simulink model "vehicle_model_999"  (R2025b)
settings: Solver=ode23tb  StartTime=0.0  StopTime=50  MaxStep=0.001  RelTol=1e-3
values from neighbouring files (symbols this model uses):
  aero_par = struct()    [Load_aero_parameters.m]
  init_r = 0    [Run_this_first.m]
  init_vx = 0    [Run_this_first.m]
  init_vy = 0    [Run_this_first.m]
  m = Par.m    [LapSim_Endurance_final_ts_v2.m]    (also in Lap_Sim_Final_inverse.m = Par.Mass; Lapsim_Endurance_final_ts.m; New_LapSim_final_ts_v1.m = Par.Mass; Torque_vectoring_lookup_table_v3.m = 270)
  Par = struct()    [Load_vehicle_parameters.m]
  sus_par = struct()    [Load_sus_parameters.m]
  TireData = []    [Lapsim_final_for_app.m]
  V_ref = 45    [Run_this_first.m]
undefined symbols (not defined in the file or in its folder): Battery, Brake_Val, HP, Ki_data, Kp_data, Motor, steer_input, Steer_Val, TC_target_slip, Throttle_Val, vx_breakpoints
libraries: simulink x7, autolibshared x2, BatteryEstimators x1
(part 1 of 3)
settings Model: Creator=vishal bhujbal  LastModifiedBy=vishal bhujbal
settings SolverCC: ZeroCrossAlgorithm=Adaptive
settings DebuggingCC: IgnoredZcDiagnostic=none

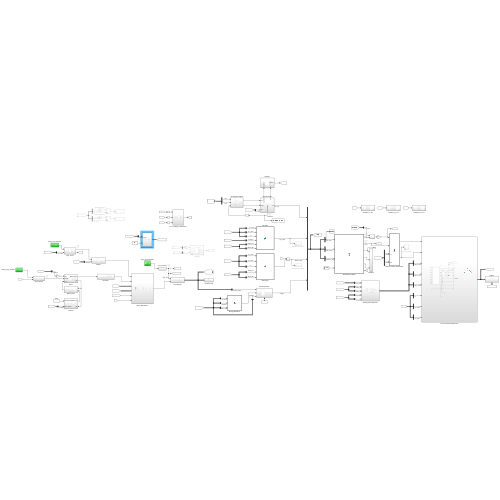
[thumbnail: Simulink's stored preview of the top-level diagram]
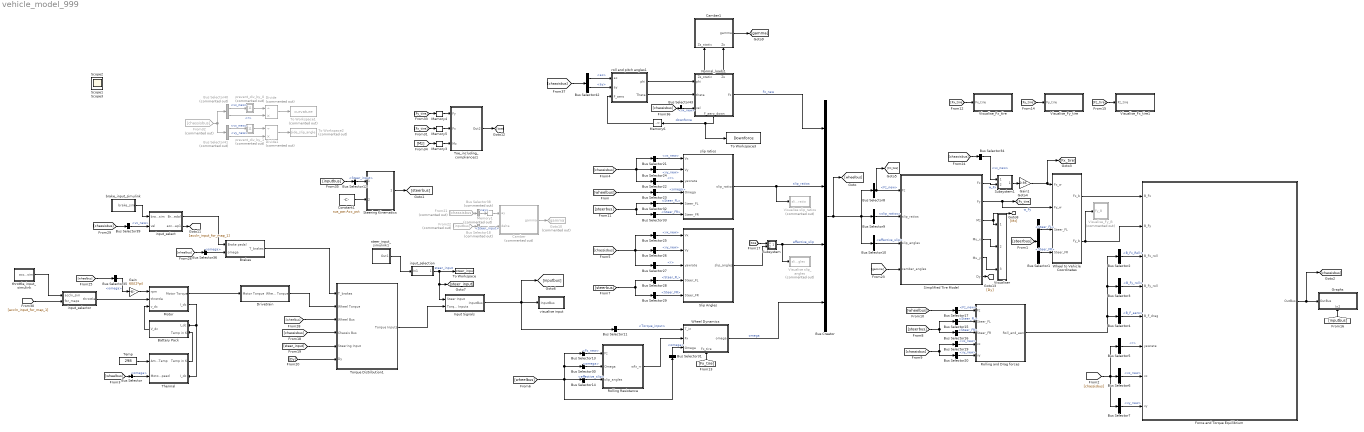
== system vehicle_model_999 ==
  Battery Pack : Subsystem
  Brakes : Subsystem
  Bus Creator : BusCreator  Inputs=4
  Bus Selector{,23,30..31,35..36} (6 alike) : BusSelector  OutputSignals=omega
  Bus Selector1 : BusSelector  OutputSignals=Steer_FL,Steer_FR
  Bus Selector10 : BusSelector  OutputSignals=effective_slip
  Bus Selector11 : BusSelector  OutputSignals=Torque_input
  Bus Selector12 : BusSelector  OutputSignals=Steer_input
  Bus Selector13 : BusSelector  OutputSignals=Fz_new
  Bus Selector14 : BusSelector  OutputSignals=effective_slip
  Bus Selector15 : BusSelector  OutputSignals=Steer_FL
  Bus Selector16 : BusSelector  OutputSignals=Steer_FR
  Bus Selector17 : BusSelector  OutputSignals=Fz_new
  Bus Selector18 : BusSelector  Commented=on  OutputSignals=Steer_input
  Bus Selector{6,19,21,25,34,39,43} (7 alike) : BusSelector  OutputSignals=vx_new
  Bus Selector2 : BusSelector  OutputSignals=B_Fx_Roll
  Bus Selector{7,20,24,26} (4 alike) : BusSelector  OutputSignals=vy_new
  Bus Selector22 : BusSelector  OutputSignals=r
  Bus Selector27 : BusSelector  OutputSignals=r
  Bus Selector28 : BusSelector  OutputSignals=Steer_FL
  Bus Selector29 : BusSelector  OutputSignals=Steer_FR
  Bus Selector3 : BusSelector  OutputSignals=B_Fy_roll
  Bus Selector32 : BusSelector  OutputSignals=Steer_FL
  Bus Selector33 : BusSelector  OutputSignals=Steer_FR
  Bus Selector38 : BusSelector  Commented=on  OutputSignals=ay
  Bus Selector4 : BusSelector  OutputSignals=B_F_aero
  Bus Selector40 : BusSelector  Commented=on  OutputSignals=vx_new,r
  Bus Selector41 : BusSelector  Commented=on  OutputSignals=vx_new,vy_new
  Bus Selector42 : BusSelector  OutputSignals=ax,ay
  Bus Selector5 : BusSelector  OutputSignals=r
  Bus Selector8 : BusSelector  OutputSignals=Fz_new
  Bus Selector9 : BusSelector  OutputSignals=slip_ratios
  Camber : Subsystem  Commented=on
  Camber1 : Subsystem
      settings: PortSchema="{\"entries\":[{\"content\":{\"sides\":[{\"content\":{},\"type\":\"ConnectorPlacement.EquallySpacedRectSide\",\"uuid\":\"3195d381-be28-49da-8fb0-abb81acde47d\"},{\"content\":{\"connectorIds\":[\"Out1\"],\"side\":\"RIGHT\"},\"type\":\"ConnectorPlacement.EquallySpacedRectSide\",\"uuid\":\"ee555968-c3bd-4b66-9d31-d91577019264\"},{\"content\":{\"side\":\"TOP\"},\"type\":\"ConnectorPlacement.EquallySpacedRectSide\",\"uuid\":\"4eacfe39-9434-48f3-a8a4-10327827cbf3\"},{\"content\":{\"connectorIds\":[\"In1\",\"In2\"],\"side\":\"BOTTOM\"},\"type\":\"ConnectorPlacement.EquallySpacedRectSide\",\"uuid\":\"1ccd728a-99da-4160-890d-6a6cfd29e494\"}]},\"type\":\"ConnectorPlacement.EquallySpacedConnector\",\"uuid\":\"ab2607e9-2e18-4a39-9990-bbd46a8a23e6\"}],\"packageUris\":[\"http://schema.mathworks.com/mf0/Connector/R2020b\"],\"version\":\"1.0\"}"
  Constant1 : Constant  Value=sus_par.Acc_pct
  Divide : Product  Commented=on  Inputs=/*
  Divide1 : Product  Commented=on  Inputs=/*
  Drivetrain : Subsystem
  Force and Torque Equilibrium : Subsystem
  From21 : From  Commented=on  GotoTag=chassisbus
  From22 : From  Commented=on  GotoTag=inputbus
  From32 : From  Commented=on  GotoTag=chassisbus
  Gain : Gain  Gain=60/(2*pi)
  Gain1 : Gain  Gain=0.95
  Goto10 : Goto  Commented=on  GotoTag=gamma
  Graphs : Subsystem
      settings: PortSchema="{\"entries\":[{\"content\":{\"sides\":[{\"content\":{\"connectorIds\":[\"In1\"]},\"type\":\"ConnectorPlacement.EquallySpacedRectSide\",\"uuid\":\"0d7f1a6c-503e-4c9f-90e9-70f717dd7dfc\"},{\"content\":{\"side\":\"RIGHT\"},\"type\":\"ConnectorPlacement.EquallySpacedRectSide\",\"uuid\":\"62097468-b066-4e29-8f99-7427d14bee77\"},{\"content\":{\"side\":\"TOP\"},\"type\":\"ConnectorPlacement.EquallySpacedRectSide\",\"uuid\":\"2a3f381e-a201-4804-99b7-77b73504b102\"},{\"content\":{\"connectorIds\":[\"In2\"],\"side\":\"BOTTOM\"},\"type\":\"ConnectorPlacement.EquallySpacedRectSide\",\"uuid\":\"dae5de0a-879c-4844-a347-7056417d054f\"}]},\"type\":\"ConnectorPlacement.EquallySpacedConnector\",\"uuid\":\"aa2835d0-6748-4566-adf9-84e8214dd5a8\"}],\"packageUris\":[\"http://schema.mathworks.com/mf0/Connector/R2020b\"],\"version\":\"1.0\"}"
  Input Signals : Subsystem
  Memory1 : Memory  Commented=on
  Memory3 : Memory
  Memory4 : Memory
  Memory5 : Memory
  Memory6 : Memory  InheritSampleTime=on
  Motor : Subsystem
  Normal_loads1 : Subsystem
      settings: PortSchema="{\"entries\":[{\"content\":{\"sides\":[{\"content\":{\"connectorIds\":[\"In1\",\"In2\",\"In3\"]},\"type\":\"ConnectorPlacement.EquallySpacedRectSide\",\"uuid\":\"5b7db607-33bd-4d54-b958-3aa960e46147\"},{\"content\":{\"connectorIds\":[\"Out1\"],\"side\":\"RIGHT\"},\"type\":\"ConnectorPlacement.EquallySpacedRectSide\",\"uuid\":\"c12df481-c511-4c4c-afb1-8a5812ce44a5\"},{\"content\":{\"connectorIds\":[\"Out3\",\"Out4\"],\"side\":\"TOP\"},\"type\":\"ConnectorPlacement.EquallySpacedRectSide\",\"uuid\":\"2c6024fe-fe45-4ba9-a61f-594b86562523\"},{\"content\":{\"connectorIds\":[\"Out2\"],\"side\":\"BOTTOM\"},\"type\":\"ConnectorPlacement.EquallySpacedRectSide\",\"uuid\":\"099189a9-186d-4ac0-a0af-1ec3a070ea03\"}]},\"type\":\"ConnectorPlacement.EquallySpacedConnector\",\"uuid\":\"81c2e338-68e5-401a-bb4f-0a973fbf41e6\"}],\"packageUris\":[\"http://schema.mathworks.com/mf0/Connector/R2020b\"],\"version\":\"1.0\"}"
  Rolling Resistance : MATLAB Function  TreatAsAtomicUnit=on
  Rolling and Drag forces : Subsystem
  Simplified Tire Model : MATLAB Function  TreatAsAtomicUnit=on
  Slip Angles : MATLAB Function  TreatAsAtomicUnit=on
  Steering Kinematics : Subsystem
  Subsystem : Subsystem
  Subsystem1 : Subsystem
  Temp : Constant  Value=298
  Thermal : Subsystem
      settings: PortSchema="{\"entries\":[{\"content\":{\"sides\":[{\"content\":{\"connectorIds\":[\"In1\",\"In2\"]},\"type\":\"ConnectorPlacement.EquallySpacedRectSide\",\"uuid\":\"a459bc8b-3545-425c-aaae-78f1ff6585f2\"},{\"content\":{\"connectorIds\":[\"Out1\",\"In3\"],\"side\":\"RIGHT\"},\"type\":\"ConnectorPlacement.EquallySpacedRectSide\",\"uuid\":\"31a206fc-68ac-4231-a8cf-74658368026e\"},{\"content\":{\"side\":\"TOP\"},\"type\":\"ConnectorPlacement.EquallySpacedRectSide\",\"uuid\":\"62e9ed2c-7fdb-44da-8c66-64d12a4ececa\"}]},\"type\":\"ConnectorPlacement.EquallySpacedConnector\",\"uuid\":\"e39d97fd-83d5-4a03-8b08-8c3e142a294f\"}],\"packageUris\":[\"http://schema.mathworks.com/mf0/Connector/R2020b\"],\"version\":\"1.0\"}"
  To Workspace : ToWorkspace  VariableName=steer_input  SaveFormat=Timeseries  SampleTime=-1
  To Workspace1 : ToWorkspace  Commented=on  VariableName=curvature  SaveFormat=Timeseries  SampleTime=-1
  To Workspace2 : ToWorkspace  Commented=on  VariableName=side_slip_angle  SaveFormat=Timeseries  SampleTime=-1
  To Workspace3 : ToWorkspace  VariableName=Downforce  SaveFormat=Timeseries  SampleTime=-1
  Toe_including_compliances1 : Subsystem
  Torque Distribution1 : Subsystem
  Visualise slip_angles : Subsystem  Commented=on
  Visualise slip_ratios : Subsystem  Commented=on
  Visualise_Fx_tire : Subsystem
  Visualise_Fx_tire1 : Subsystem
  Visualise_Fy_B : Subsystem  Commented=on
  Visualise_Fy_tire : Subsystem
  Visualiser : Subsystem
  Wheel Dynamics : Subsystem
      settings: PortSchema="{\"entries\":[{\"content\":{\"sides\":[{\"content\":{\"connectorIds\":[\"In1\",\"In2\",\"In3\"]},\"type\":\"ConnectorPlacement.EquallySpacedRectSide\",\"uuid\":\"f2e918e6-c6f6-4ec9-89f3-e2543a6374fd\"},{\"content\":{\"connectorIds\":[\"Out1\"],\"side\":\"RIGHT\"},\"type\":\"ConnectorPlacement.EquallySpacedRectSide\",\"uuid\":\"be700f5f-5cf3-4eec-a6f7-872bb7cd40f6\"},{\"content\":{\"side\":\"TOP\"},\"type\":\"ConnectorPlacement.EquallySpacedRectSide\",\"uuid\":\"c4f49273-9888-4d11-a98e-35dc6f585916\"},{\"content\":{\"connectorIds\":[\"In4\"],\"side\":\"BOTTOM\"},\"type\":\"ConnectorPlacement.EquallySpacedRectSide\",\"uuid\":\"8d2e7982-4362-4abb-b8fe-c155beeed1bc\"}]},\"type\":\"ConnectorPlacement.EquallySpacedConnector\",\"uuid\":\"4d6dafa1-905e-4e38-a48b-73a98e690073\"}],\"packageUris\":[\"http://schema.mathworks.com/mf0/Connector/R2020b\"],\"version\":\"1.0\"}"
  Wheel to Vehicle Coordinates : MATLAB Function  TreatAsAtomicUnit=on
  brake_input_simulink : Subsystem
  input_select : Subsystem
  input_selection : Subsystem
  input_selector : Subsystem
  prevent_div_by_0 : Subsystem  Commented=on
  prevent_div_by_1 : Subsystem  Commented=on
  roll and pitch angles1 : Subsystem
  slip ratios : MATLAB Function  TreatAsAtomicUnit=on
  steer_input_simulink1 : Subsystem
  throttle_input_simulink : Subsystem
  visualise input : Subsystem
  Scope1 : Scope
      settings: ActiveDisplayYMinimum=-36.556875  ActiveDisplayYMaximum=329.01187500000003  DataLoggingVariableName=ScopeData7
  Scope2 : Scope
      settings: ActiveDisplayYMinimum=-33.26675625  ActiveDisplayYMaximum=299.40080625000007  DataLoggingVariableName=ScopeData9
  Scope3 : Scope
      settings: ActiveDisplayYMinimum=-1  ActiveDisplayYMaximum=1  DataLoggingVariableName=ScopeData10
  wires:
  [toe] -> Subsystem/1(toe)
  [Fy_tire] -> Visualise_Fy_tire/1(Fy_tire)
  From22/1 -> Bus Selector18/1
  Bus Selector33/1 -> slip ratios/6(Steer_FR)  "<Steer_FR>"
  Subsystem/1(Out1) -> Bus Creator/3, Visualise slip_angles/1(slip_angles)  "effective_slip"
  Bus Selector41/2 -> Divide1/2  "<vy_new>"
  Bus Selector15/1 -> Rolling and Drag forces/2(Steer_FL)  "<Steer_FL>"
  [wheelbus] -> Bus Selector35/1
  Input Signals/1(InputBus) -> [inputbus], visualise input/1(InputBus), Bus Selector11/1
  [chassisbus] -> Bus Selector27/1, Bus Selector26/1, Bus Selector25/1
  input_select/2(accln_for_map1) -> [accln_input_for_map_1]
  Bus Selector41/1 -> prevent_div_by_1/1(In1)  "<vx_new>"
  Bus Selector1/1 -> Wheel to Vehicle Coordinates/3(Steer_FL)  "<Steer_FL>"
  Motor/1(Motor Torque) -> Drivetrain/1(Motor Torque)
  Bus Selector27/1 -> Slip Angles/3(yawrate)  "<r>"
  [steerbus] -> Bus Selector33/1, Bus Selector32/1
  Simplified Tire Model/2(Fy) -> Wheel to Vehicle Coordinates/2(Fy_w), [Fy_tire]  "w_Fy"
  Bus Selector11/1 -> Wheel Dynamics/1(T_in)  "<Torque_input>"
  prevent_div_by_0/1(Out1) -> Divide/1
  Bus Selector26/1 -> Slip Angles/2(Vy)  "<vy_new>"
  [inputbus] -> Graphs/2(In2)
  Bus Selector14/1 -> Rolling Resistance/3(slip_angles)  "<effective_slip>"
  [chassisbus] -> Bus Selector39/1
  Bus Selector25/1 -> Slip Angles/1(Vx)  "<vx_new>"
  Temp/1 -> Thermal/1(Ambient Temp)
  [accln_input_for_map_1] -> input_selector/2(for_maps)
  Bus Selector30/1 -> Rolling Resistance/2(Omega)  "<omega>"
  Gain/1 -> Motor/1(rpm)
  Divide/1 -> To Workspace1/1
  Rolling and Drag forces/1(Roll_and_aero) -> Bus Selector2/1, Bus Selector3/1, Bus Selector4/1
  Bus Selector20/1 -> Rolling and Drag forces/5(vy)  "<vy_new>"
  input_selection/1(Steer Input) -> Input Signals/1(Steer Input), [steer_input], To Workspace/1  "steer_input"
  [steerbus] -> Bus Selector1/1
  Simplified Tire Model/4(Mu_x) -> Visualiser/2(mu_x)
  Force and Torque Equilibrium/1(OutBus) -> Graphs/1(OutBus), [chassisbus]
  Drivetrain/1(Wheel Torque) -> Torque Distribution1/2(Wheel Torque)
  Bus Selector5/1 -> Force and Torque Equilibrium/6(yawrate)  "<r>"
  Bus Selector35/1 -> Gain/1  "<omega>"
  Rolling Resistance/1(wFx_rr) -> Wheel Dynamics/2(Fx)
  Bus Selector18/1 -> Camber/2(delta)  "<Steer_input>"
  Bus Selector24/1 -> slip ratios/2(Vy)  "<vy_new>"
  Bus Selector9/1 -> Simplified Tire Model/2(slip_ratios)  "<slip_ratios>"
  Bus Creator/1 -> Bus Selector10/1, Bus Selector8/1, Bus Selector9/1, [wheelbus]
  [chassisbus] -> Bus Selector34/1
  Camber/1(gamma) -> Goto10/1
  Battery Pack/1(V_dc) -> Motor/3(v_dc)
  Bus Selector16/1 -> Rolling and Drag forces/3(Steer_FR)  "<Steer_FR>"
  Bus Selector22/1 -> slip ratios/3(yawrate)  "<r>"
  Bus Selector17/1 -> Rolling and Drag forces/1(Fz)  "<Fz_new>"
  [gamma] -> Simplified Tire Model/4(camber_angles)
  [chassisbus] -> Bus Selector22/1, Bus Selector24/1, Bus Selector21/1
  [steerbus] -> Bus Selector29/1, Bus Selector28/1
  Bus Selector10/1 -> Simplified Tire Model/3(slip_angles)  "<effective_slip>"
  input_select/1(Brake pedal) -> Brakes/1(Brake pedal)
  Bus Selector39/1 -> input_select/2(vel)  "<vx_new>"
  Bus Selector19/1 -> Rolling and Drag forces/4(vx)  "<vx_new>"
  [wheelbus] -> Bus Selector13/1, Bus Selector30/1, Bus Selector14/1, Bus Selector31/1
  Bus Selector12/1 -> Steering Kinematics/1(Steer_Input)  "<Steer_input>"
  [wheelbus] -> Bus Selector36/1
  Bus Selector8/1 -> [Fz_tire], Simplified Tire Model/1(Fz)  "<Fz_new>"
  [wheelbus] -> Bus Selector23/1
  [wheelbus] -> Bus Selector17/1
  [Fz_tire] -> Visualise_Fx_tire1/1(Fz_tire)
  Bus Selector40/1 -> prevent_div_by_0/1(In1)  "<vx_new>"
  [Fx_tire] -> Visualise_Fx_tire/1(Fx_tire)
  Bus Selector28/1 -> Slip Angles/4(Steer_FL)  "<Steer_FL>"
  Divide1/1 -> To Workspace2/1
  slip ratios/1(slip_ratios) -> Visualise slip_ratios/1(slip_ratio), Bus Creator/2  "slip_ratios"
  Bus Selector3/1 -> Force and Torque Equilibrium/4(B_Fy_roll)  "<B_Fy_roll>"
  Bus Selector40/2 -> Divide/2  "<r>"
  [inputbus] -> Bus Selector12/1
  Bus Selector21/1 -> slip ratios/1(Vx)  "<vx_new>"
  Brakes/1(T_brakes) -> Torque Distribution1/1(T_brakes)
  Simplified Tire Model/5(Mu_y) -> Visualiser/3(mu_y)
  [chassisbus] -> Bus Selector5/1, Bus Selector6/1, Bus Selector7/1
  Wheel Dynamics/1(omega) -> Bus Creator/4  "omega"
  Slip Angles/1(slip_angles) -> Subsystem/2(slip_angles)
  Bus Selector32/1 -> slip ratios/5(Steer_FL)  "<Steer_FL>"
  Torque Distribution1/1(Torque Inputs) -> Input Signals/2(Torque Inputs)
  Bus Selector34/1 -> Subsystem1/1(Vx)  "<vx_new>"
  input_selector/1(throttle) -> Motor/2(throttle)
  Subsystem1/1(Fx_w) -> Gain1/1
  Bus Selector6/1 -> Force and Torque Equilibrium/7(vx)  "<vx_new>"
  Motor/2(I_dc) -> Thermal/3(I_dc), Battery Pack/1(I_dc)
  Thermal/1(Temp in K) -> Battery Pack/2(Temp in K)
  Bus Selector4/1 -> Force and Torque Equilibrium/5(B_F_drag)  "<B_F_aero>"
  [Fx_tire] -> Wheel Dynamics/4(Fx_tire)
  Wheel to Vehicle Coordinates/2(Fy_b) -> Visualise_Fy_B/1(Fy_B), Force and Torque Equilibrium/2(B_Fy)
  [chassisbus] -> Bus Selector19/1, Bus Selector20/1
  From32/1 -> Bus Selector40/1, Bus Selector41/1
  Bus Selector29/1 -> Slip Angles/5(Steer_FR)  "<Steer_FR>"
  [steerbus] -> Bus Selector15/1, Bus Selector16/1
  Bus Selector13/1 -> Rolling Resistance/1(Fz)  "<Fz_new>"
  Bus Selector36/1 -> Brakes/2(omega)  "<omega>"
  Bus Selector31/1 -> Wheel Dynamics/3(Omega)  "<omega>"
  Toe_including_compliances1/1(Out2) -> [toe]
  [Fx_tire] -> Memory5/1
  [Mz] -> Memory3/1
  steer_input_simulink1/1(Out1) -> input_selection/1(In1)
  [Fy_tire] -> Memory4/1
  Constant1/1 -> Steering Kinematics/2(Ackermann_Pct)
  Bus Selector2/1 -> Force and Torque Equilibrium/3(B_Fx_roll)  "<B_Fx_Roll>"
  Bus Selector7/1 -> Force and Torque Equilibrium/8(vy)  "<vy_new>"
  brake_input_simulink/1(brake_sim) -> input_select/1(brake_sim)
  Steering Kinematics/1(Steering Angles) -> [steerbus]
  Bus Selector23/1 -> slip ratios/4(Omega)  "<omega>"
  Bus Selector1/2 -> Wheel to Vehicle Coordinates/4(Steer_FR)  "<Steer_FR>"
  Simplified Tire Model/1(Fx) -> Subsystem1/2(Fx_ss)  "w_Fx"
  [wheelbus] -> Torque Distribution1/3(Wheel Bus)
  [chassisbus] -> Torque Distribution1/4(Chassis Bus)
  [steer_input] -> Torque Distribution1/5(Steering Input)
  Simplified Tire Model/6(Dy) -> [Dy]
  [Dy] -> Torque Distribution1/6(Dy)
  prevent_div_by_1/1(Out1) -> Divide1/1
  Memory4/1 -> Toe_including_compliances1/1(Fy)
  Gain1/1 -> [Fx_tire], Wheel to Vehicle Coordinates/1(Fx_w)
  Wheel to Vehicle Coordinates/1(Fx_b) -> Force and Torque Equilibrium/1(B_Fx)
  Memory5/1 -> Toe_including_compliances1/2(Fx)
  Simplified Tire Model/3(Mz) -> Visualiser/1(mz), [Mz]
  From21/1 -> Bus Selector38/1
  Bus Selector38/1 -> Memory1/1  "<ay>"
  Memory1/1 -> Camber/1(ay)
  Memory3/1 -> Toe_including_compliances1/3(Mz)
  roll and pitch angles1/1(phi) -> Normal_loads1/1(phi)
  Bus Selector42/1 -> roll and pitch angles1/1(ax)  "<ax>"
  [chassisbus] -> Bus Selector43/1
  Bus Selector43/1 -> Normal_loads1/3(vel)  "<vx_new>"
  Memory6/1 -> roll and pitch angles1/3(F_aero)
  Normal_loads1/1(Fz) -> Bus Creator/1  "Fz_new"
  Normal_loads1/2(F_aero_down) -> To Workspace3/1, Memory6/1  "downforce"
  roll and pitch angles1/2(Theta) -> Normal_loads1/2(theta)
  Camber1/1(gamma) -> [gamma]
  [chassisbus] -> Bus Selector42/1
  Normal_loads1/3(Zs_static) -> Camber1/1(Zs_static)
  Normal_loads1/4(Zs) -> Camber1/2(Zs)
  Bus Selector42/2 -> roll and pitch angles1/2(ay)  "<ay>"
  throttle_input_simulink/1(accln_sim) -> input_selector/1(accln_sim)
  [wheelbus] -> Bus Selector/1
  Bus Selector/1 -> Thermal/2(Motor speed)  "<omega>"

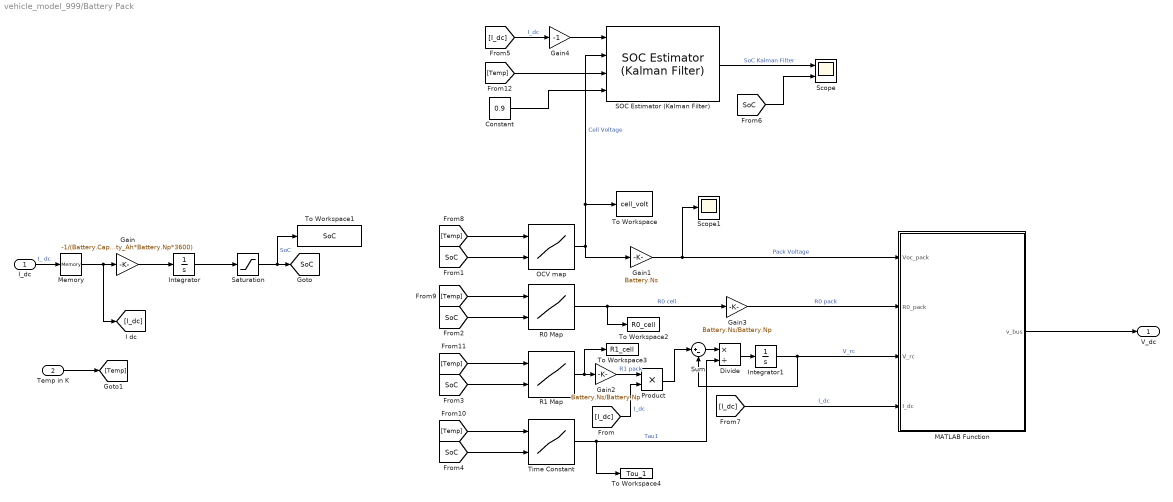
== system vehicle_model_999/Battery Pack ==
  I_dc : Inport
  Temp in K : Inport  Port=2
  Constant : Constant  Value=0.9
  Divide : Product  Inputs=*/
  Gain : Gain  Gain=-1/(Battery.Capacity_Ah*Battery.Np*3600)
  Gain1 : Gain  Gain=Battery.Ns
  Gain2 : Gain  Gain=Battery.Ns/Battery.Np
  Gain3 : Gain  Gain=Battery.Ns/Battery.Np
  Gain4 : Gain  Gain=-1
  Integrator : Integrator  InitialCondition=1
  Integrator1 : Integrator
  MATLAB Function : MATLAB Function  TreatAsAtomicUnit=on
  Memory : Memory
  OCV map : Lookup_n-D  BreakpointsForDimension1=Battery.T_vec  BreakpointsForDimension2=Battery.SoC_vec  Table=Battery.OCV_map'  InternalRulePriority=Speed  RndMeth=Simplest
      settings: InputPortMap=u0,u1
  Product : Product
  R0 Map : Lookup_n-D  BreakpointsForDimension1=Battery.T_vec  BreakpointsForDimension2=Battery.SoC_vec  Table=Battery.R0_map'  InternalRulePriority=Speed  RndMeth=Simplest
      settings: InputPortMap=u0,u1
  R1 Map : Lookup_n-D  BreakpointsForDimension1=Battery.T_vec  BreakpointsForDimension2=Battery.SoC_vec  Table=Battery.R1_map'  InternalRulePriority=Speed  RndMeth=Simplest
      settings: InputPortMap=u0,u1
  SOC Estimator (Kalman Filter) : BatteryEstimators/SOC Estimator (Kalman Filter)  CurrentInputPartition=off  filterType=Extended Kalman filter  alpha=1  beta=2  kappa=0  Q=|  Q_2RC=|  R=0.1  P0=[1e-5 0; 0 1]  P0_2RC=[1e-5 0 0; 0 1 0;0 0 1]  Ts=1  chargeDynamics=One time-constant dynamics  SOC_vec=[0 0.1 0.25 0.5 0.75 0.9 1]  T_vec=[278 293 313]  R0_mat=[0.0117 0.0085 0.009;0.011 0.0085 0.009;0.0114 0.0087 0.0092;0.0107 0.0082 0.0088;0.0107 0.0083 0.0091;0.0113 0.0085 0.0089;0.0116 0.0085 0.0089]  R1_mat=[0.0109 0.0029 0.0013;0.0069 0.0024 0.0012;0.0047 0.0026 0.0013;0.0034 0.0016 0.001;0.0033 0.0023 0.0014;0.0033 0.0018 0.0011;0.0028 0.0017 0.0011]  tau1_mat=[20 36 39;31 45 39;109 105 61;36 29 26;59 77 67;40 33 29;25 39 33]  R2_mat=[.0109, .0029, .0013; .0069, .0024, .0012; .0047, .0026, .0013; .0034, .0016, .001; .0033, .0023, .0014; .0033, .0018, .0011; .0028, .0017, .0011]  tau2_mat=[20, 36, 39; 31, 45, 39; 109, 105, 61; 36, 29, 26; 59, 77, 67; 40, 33, 29; 25, 39, 33]  V0_mat=[3.49 3.5 3.51;3.55 3.57 3.56;3.62 3.63 3.64;3.71 3.71 3.72;3.91 3.93 3.94;4.07 4.08 4.08;4.19 4.19 4.19]  AH=4.493  DataType=Inherit: auto
      Q=|
      | [1e-6 0;
      | 0 1e-6]
      Q_2RC=|
      | [1e-6 0 0;
      | 0 1e-6 0; 0 0 1e-6]
  Saturation : Saturate  UpperLimit=1  LowerLimit=0
  Scope : Scope  NumInputPorts=2
      settings: ActiveDisplayYMinimum=0.74078  ActiveDisplayYMaximum=0.86214  DataLoggingVariableName=ScopeData8
  Scope1 : Scope
      settings: ActiveDisplayYMinimum=583.0264  ActiveDisplayYMaximum=588.0193  DataLoggingVariableName=ScopeData14
  Sum : Sum  Inputs=|+-
  Time Constant : Lookup_n-D  BreakpointsForDimension1=Battery.T_vec  BreakpointsForDimension2=Battery.SoC_vec  Table=Battery.Tau_map'  InternalRulePriority=Speed  RndMeth=Simplest
      settings: InputPortMap=u0,u1
  To Workspace : ToWorkspace  VariableName=cell_volt  SaveFormat=Timeseries  SampleTime=-1
  To Workspace1 : ToWorkspace  VariableName=SoC  SaveFormat=Timeseries  SampleTime=-1
  To Workspace2 : ToWorkspace  VariableName=R0_cell  SaveFormat=Timeseries  SampleTime=-1
  To Workspace3 : ToWorkspace  VariableName=R1_cell  SaveFormat=Timeseries  SampleTime=-1
  To Workspace4 : ToWorkspace  VariableName=Tou_1  SaveFormat=Timeseries  SampleTime=-1
  V_dc : Outport
  tag scope: SoC=global
  wires:
  I_dc/1 -> Memory/1  "I_ dc"
  Gain/1 -> Integrator/1
  Integrator/1 -> Saturation/1
  OCV map/1 -> SOC Estimator (Kalman Filter)/2, To Workspace/1, Gain1/1  "Cell Voltage"
  Gain1/1 -> Scope1/1, MATLAB Function/1(Voc_pack)  "Pack Voltage"
  R1 Map/1 -> To Workspace3/1, Gain2/1
  R0 Map/1 -> To Workspace2/1, Gain3/1  "R0 cell"
  Gain3/1 -> MATLAB Function/2(R0_pack)  "R0 pack"
  Gain2/1 -> Product/1  "R1 pack"
  Product/1 -> Sum/1
  Integrator1/1 -> MATLAB Function/3(V_rc), Sum/2  "V_rc"
  Sum/1 -> Divide/1
  Time Constant/1 -> To Workspace4/1, Divide/2  "Tau1"
  Divide/1 -> Integrator1/1
  Constant/1 -> SOC Estimator (Kalman Filter)/4
  SOC Estimator (Kalman Filter)/1 -> Scope/1  "SoC Kalman Filter"
  MATLAB Function/1(v_bus) -> V_dc/1
  [I_dc] -> Product/2  "I_dc"
  Saturation/1 -> To Workspace1/1, [SoC]  "SoC"
  [SoC] -> Time Constant/2
  [SoC] -> R1 Map/2
  [SoC] -> R0 Map/2
  [SoC] -> OCV map/2
  [I_dc] -> Gain4/1  "I_dc"
  [SoC] -> Scope/2
  [I_dc] -> MATLAB Function/4(I_dc)  "I_dc"
  Temp in K/1 -> [Temp]
  [Temp] -> OCV map/1
  [Temp] -> R0 Map/1
  [Temp] -> R1 Map/1
  [Temp] -> Time Constant/1
  [Temp] -> SOC Estimator (Kalman Filter)/3
  Memory/1 -> [I_dc], Gain/1
  Gain4/1 -> SOC Estimator (Kalman Filter)/1

== system vehicle_model_999/Brakes ==
  Brake pedal : Inport
  omega : Inport  Port=2
  Gain : Gain  Gain=100
  MATLAB Function : MATLAB Function  TreatAsAtomicUnit=on
  Terminator : Terminator
  Terminator1 : Terminator
  Terminator2 : Terminator
  To Workspace : ToWorkspace  VariableName=brk_ipt_pct  SaveFormat=Timeseries  SampleTime=-1
  To Workspace1 : ToWorkspace  VariableName=Front_braking_torque  SaveFormat=Timeseries  SampleTime=-1
  To Workspace2 : ToWorkspace  VariableName=Rear_braking_torque  SaveFormat=Timeseries  SampleTime=-1
  T_brakes : Outport
  wires:
  MATLAB Function/1(T_brakes) -> T_brakes/1
  omega/1 -> MATLAB Function/2(omega)
  Brake pedal/1 -> Gain/1, MATLAB Function/1(brake_pedal)  "Brake_input"
  MATLAB Function/2(T_mag_Front) -> Terminator/1, To Workspace1/1  "Front_braking_torque"
  MATLAB Function/3(T_mag_Rear) -> To Workspace2/1, Terminator1/1  "Rear_braking_torque"
  Gain/1 -> Terminator2/1, To Workspace/1  "brak_pedal_input_percent"

== system vehicle_model_999/Camber ==
  ay : Inport
  delta : Inport  Port=2
  MATLAB Function : MATLAB Function  TreatAsAtomicUnit=on
  Mux : Mux
  gamma : Outport
  wires:
  MATLAB Function/1(gamma_FR) -> Mux/1
  MATLAB Function/2(gamma_FL) -> Mux/2
  MATLAB Function/3(gamma_RL) -> Mux/3
  MATLAB Function/4(gamma_RR) -> Mux/4
  Mux/1 -> gamma/1
  ay/1 -> MATLAB Function/1(ay)
  delta/1 -> MATLAB Function/2(delta)

== system vehicle_model_999/Camber1 ==
  Zs_static : Inport
  Zs : Inport  Port=2
  DynamicCamber_FromHP_Zmeters : MATLAB Function  TreatAsAtomicUnit=on
  Subsystem : Subsystem
  Subsystem1 : Subsystem  Commented=on
  Subsystem2 : Subsystem  Commented=on
  gamma : Outport
  wires:
  DynamicCamber_FromHP_Zmeters/1(Camber) -> gamma/1, Subsystem/1(Camber)
  Zs/1 -> DynamicCamber_FromHP_Zmeters/1(Zs)
  Zs_static/1 -> DynamicCamber_FromHP_Zmeters/2(Zs_static)
  DynamicCamber_FromHP_Zmeters/2(dynamic_camber_visualisation) -> Subsystem1/1(dynamic_camber)
  DynamicCamber_FromHP_Zmeters/3(static_camber_visualisation) -> Subsystem2/1(static_camber)

== system vehicle_model_999/Drivetrain ==
  Motor Torque : Inport
  Demux : Demux  Outputs=2
  Gear Ratio : Gain  Gain=Motor.gear_ratio
  MATLAB Function : MATLAB Function  TreatAsAtomicUnit=on
  Mux : Mux
  Overall Powertrain Efficiency : Gain  Gain=Motor.overall_efficiency
  Wheel Torque : Outport
  wires:
  Motor Torque/1 -> Gear Ratio/1
  Gear Ratio/1 -> Overall Powertrain Efficiency/1
  MATLAB Function/1(T_fl) -> Mux/1
  MATLAB Function/2(T_fr) -> Mux/2
  Demux/1 -> Mux/3
  Demux/2 -> Mux/4
  Mux/1 -> Wheel Torque/1
  Overall Powertrain Efficiency/1 -> Demux/1

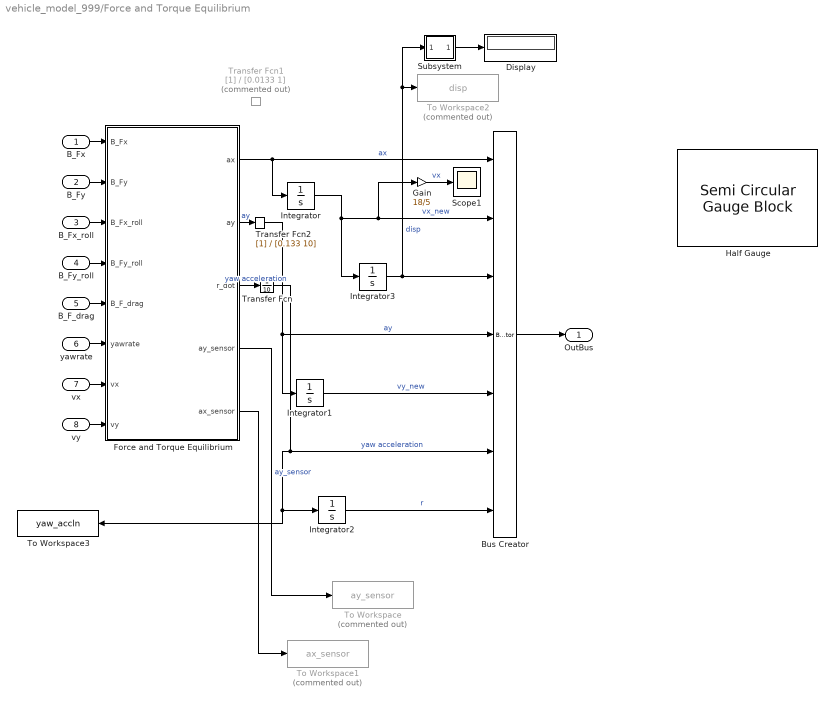
== system vehicle_model_999/Force and Torque Equilibrium ==
  B_Fx : Inport
  B_Fy : Inport  Port=2
  B_Fx_roll : Inport  Port=3
  B_Fy_roll : Inport  Port=4
  B_F_drag : Inport  Port=5
  yawrate : Inport  Port=6
  vx : Inport  Port=7
  vy : Inport  Port=8
  Bus Creator : BusCreator  Inputs=7
  Display : Display
  Force and Torque Equilibrium : MATLAB Function  TreatAsAtomicUnit=on
  Gain : Gain  Gain=18/5
  Half Gauge : SemiCircularGaugeBlock  ScaleMax=150  FontColor=[0.0, 0.0, 0.0]
  Integrator : Integrator  InitialCondition=init_vx  LimitOutput=on  UpperSaturationLimit=1e6  LowerSaturationLimit=0
  Integrator1 : Integrator  InitialCondition=init_vy  LimitOutput=on  UpperSaturationLimit=1e6
  Integrator2 : Integrator  InitialCondition=init_r  LimitOutput=on  UpperSaturationLimit=1e6
  Integrator3 : Integrator
  Scope1 : Scope
      settings: ActiveDisplayYMinimum=-1  ActiveDisplayYMaximum=1  DataLoggingVariableName=ScopeData20
  Subsystem : Subsystem
  To Workspace : ToWorkspace  Commented=on  VariableName=ay_sensor  SaveFormat=Timeseries  SampleTime=-1
  To Workspace1 : ToWorkspace  Commented=on  VariableName=ax_sensor  SaveFormat=Timeseries  SampleTime=-1
  To Workspace2 : ToWorkspace  Commented=on  VariableName=disp  SaveFormat=Timeseries  SampleTime=-1
  To Workspace3 : ToWorkspace  VariableName=yaw_accln  SaveFormat=Timeseries  SampleTime=-1
  Transfer Fcn : TransferFcn  Denominator=[0 10]
  Transfer Fcn1 : TransferFcn  Commented=on  Denominator=[0.0133 1]
  Transfer Fcn2 : TransferFcn  Denominator=[0.133 10]
  OutBus : Outport
  wires:
  Force and Torque Equilibrium/4(ay_sensor) -> To Workspace/1  "ay_sensor"
  B_Fx/1 -> Force and Torque Equilibrium/1(B_Fx)
  Integrator1/1 -> Bus Creator/5  "vy_new"
  B_F_drag/1 -> Force and Torque Equilibrium/5(B_F_drag)
  B_Fy/1 -> Force and Torque Equilibrium/2(B_Fy)
  vy/1 -> Force and Torque Equilibrium/8(vy)
  Integrator2/1 -> Bus Creator/7  "r"
  Integrator3/1 -> Subsystem/1(In1), To Workspace2/1, Bus Creator/3  "disp"
  Force and Torque Equilibrium/1(ax) -> Bus Creator/1, Integrator/1  "ax"
  Bus Creator/1 -> OutBus/1
  B_Fx_roll/1 -> Force and Torque Equilibrium/3(B_Fx_roll)
  B_Fy_roll/1 -> Force and Torque Equilibrium/4(B_Fy_roll)
  yawrate/1 -> Force and Torque Equilibrium/6(yawrate)
  Force and Torque Equilibrium/3(r_dot) -> Transfer Fcn/1  "yaw acceleration"
  Integrator/1 -> Integrator3/1, Bus Creator/2, Gain/1  "vx_new"
  vx/1 -> Force and Torque Equilibrium/7(vx)
  Force and Torque Equilibrium/5(ax_sensor) -> To Workspace1/1
  Subsystem/1(Out1) -> Display/1
  Gain/1 -> Scope1/1  "vx"
  Force and Torque Equilibrium/2(ay) -> Transfer Fcn2/1  "ay"
  Transfer Fcn/1 -> To Workspace3/1, Integrator2/1, Bus Creator/6  "yaw acceleration"
  Transfer Fcn2/1 -> Integrator1/1, Bus Creator/4  "ay"

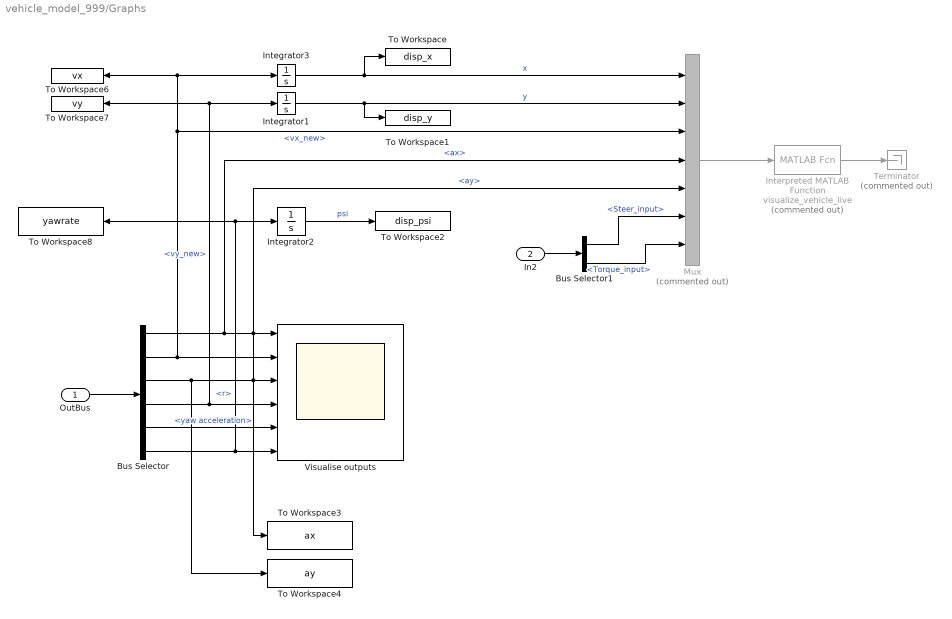
== system vehicle_model_999/Graphs ==
  OutBus : Inport
  In2 : Inport  Port=2
  Bus Selector : BusSelector  OutputSignals=ax,vx_new,ay,vy_new,yaw acceleration,r
  Bus Selector1 : BusSelector  OutputSignals=Steer_input,Torque_input
  Integrator1 : Integrator
  Integrator2 : Integrator
  Integrator3 : Integrator
  Interpreted MATLAB Function : MATLABFcn  Commented=on  MATLABFcn=visualize_vehicle_live
  Mux : Mux  Commented=on  Inputs=7
  Terminator : Terminator  Commented=on
  To Workspace : ToWorkspace  VariableName=disp_x  SaveFormat=Timeseries  SampleTime=-1
  To Workspace1 : ToWorkspace  VariableName=disp_y  SaveFormat=Timeseries  SampleTime=-1
  To Workspace2 : ToWorkspace  VariableName=disp_psi  SaveFormat=Timeseries  SampleTime=-1
  To Workspace3 : ToWorkspace  VariableName=ax  SaveFormat=Timeseries  SampleTime=-1
  To Workspace4 : ToWorkspace  VariableName=ay  SaveFormat=Timeseries  SampleTime=-1
  To Workspace6 : ToWorkspace  VariableName=vx  SaveFormat=Timeseries  SampleTime=-1
  To Workspace7 : ToWorkspace  VariableName=vy  SaveFormat=Timeseries  SampleTime=-1
  To Workspace8 : ToWorkspace  VariableName=yawrate  SaveFormat=Timeseries  SampleTime=-1
  Visualise outputs : Scope  NumInputPorts=6
      settings: ActiveDisplayYMinimum=-4.6342957634228235  ActiveDisplayYMaximum=6.3753103405334306  DataLoggingVariableName=ScopeData2
  wires:
  OutBus/1 -> Bus Selector/1
  Bus Selector/1 -> To Workspace3/1, Visualise outputs/1, Mux/4  "<ax>"
  Bus Selector/2 -> Integrator3/1, To Workspace6/1, Mux/3, Visualise outputs/2  "<vx_new>"
  Bus Selector/3 -> Mux/5, Visualise outputs/3, To Workspace4/1  "<ay>"
  Bus Selector/4 -> Integrator1/1, To Workspace7/1, Visualise outputs/4  "<vy_new>"
  Bus Selector/5 -> Visualise outputs/5  "<yaw acceleration>"
  Integrator3/1 -> Mux/1, To Workspace/1  "x"
  Integrator1/1 -> To Workspace1/1, Mux/2  "y"
  Integrator2/1 -> To Workspace2/1  "psi"
  Mux/1 -> Interpreted MATLAB Function/1
  Interpreted MATLAB Function/1 -> Terminator/1
  In2/1 -> Bus Selector1/1
  Bus Selector1/1 -> Mux/6  "<Steer_input>"
  Bus Selector1/2 -> Mux/7  "<Torque_input>"
  Bus Selector/6 -> Integrator2/1, To Workspace8/1, Visualise outputs/6  "<r>"

== system vehicle_model_999/Input Signals ==
  Steer Input : Inport
  Torque Inputs : Inport  Port=2
  Bus Creator : BusCreator  Inputs=2
  InputBus : Outport
  wires:
  Torque Inputs/1 -> Bus Creator/1  "Torque_input"
  Steer Input/1 -> Bus Creator/2  "Steer_input"
  Bus Creator/1 -> InputBus/1

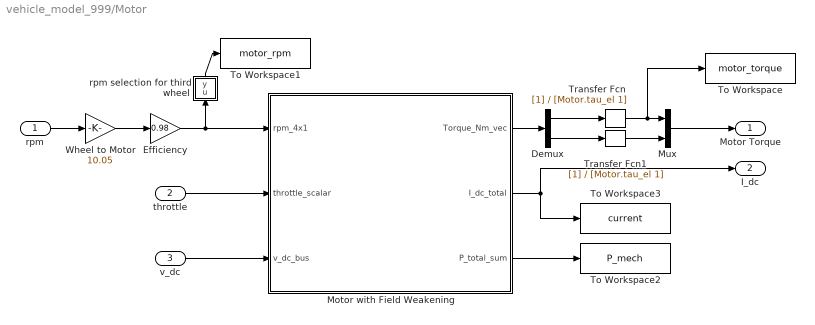
== system vehicle_model_999/Motor ==
  rpm : Inport
  throttle : Inport  Port=2
  v_dc : Inport  Port=3
  Demux : Demux  Outputs=2
  Efficiency : Gain  Gain=0.98
  Motor with Field Weakening : MATLAB Function  TreatAsAtomicUnit=on
  Mux : Mux  Inputs=2
  To Workspace : ToWorkspace  VariableName=motor_torque  SaveFormat=Timeseries  SampleTime=-1
  To Workspace1 : ToWorkspace  VariableName=motor_rpm  SaveFormat=Timeseries  SampleTime=-1
  To Workspace2 : ToWorkspace  VariableName=P_mech  SaveFormat=Timeseries  SampleTime=-1
  To Workspace3 : ToWorkspace  VariableName=current  SaveFormat=Timeseries  SampleTime=-1
  Transfer Fcn : TransferFcn  Denominator=[Motor.tau_el 1]
  Transfer Fcn1 : TransferFcn  Denominator=[Motor.tau_el 1]
  Wheel to Motor : Gain  Gain=10.05
  rpm selection for third wheel : MATLAB Function  TreatAsAtomicUnit=on
  Motor Torque : Outport
  I_dc : Outport  Port=2
  wires:
  rpm/1 -> Wheel to Motor/1
  throttle/1 -> Motor with Field Weakening/2(throttle_scalar)
  v_dc/1 -> Motor with Field Weakening/3(v_dc_bus)
  Wheel to Motor/1 -> Efficiency/1
  Efficiency/1 -> rpm selection for third wheel/1(u), Motor with Field Weakening/1(rpm_4x1)
  Motor with Field Weakening/2(I_dc_total) -> I_dc/1, To Workspace3/1
  Motor with Field Weakening/1(Torque_Nm_vec) -> Demux/1
  Demux/1 -> Transfer Fcn/1
  Transfer Fcn1/1 -> Mux/2
  Demux/2 -> Transfer Fcn1/1
  Transfer Fcn/1 -> To Workspace/1, Mux/1
  Mux/1 -> Motor Torque/1
  Motor with Field Weakening/3(P_total_sum) -> To Workspace2/1
  rpm selection for third wheel/1(y) -> To Workspace1/1

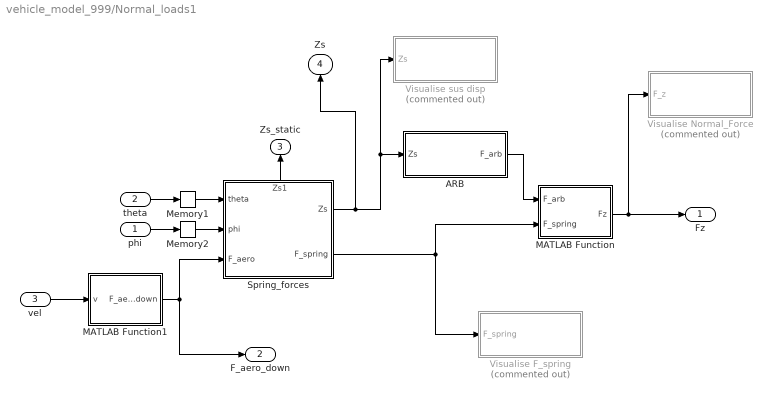
== system vehicle_model_999/Normal_loads1 ==
  phi : Inport
  theta : Inport  Port=2
  vel : Inport  Port=3
  ARB : Subsystem
  MATLAB Function : MATLAB Function  TreatAsAtomicUnit=on
  MATLAB Function1 : MATLAB Function  TreatAsAtomicUnit=on
  Memory1 : Memory
  Memory2 : Memory
  Spring_forces : Subsystem
      settings: PortSchema="{\"entries\":[{\"content\":{\"sides\":[{\"content\":{\"connectorIds\":[\"In1\",\"In2\",\"In3\"]},\"type\":\"ConnectorPlacement.EquallySpacedRectSide\",\"uuid\":\"355bde33-3e3d-4de3-a05a-1287e2d3eebd\"},{\"content\":{\"connectorIds\":[\"Out1\",\"Out2\"],\"side\":\"RIGHT\"},\"type\":\"ConnectorPlacement.EquallySpacedRectSide\",\"uuid\":\"644c8213-6936-480f-b4bc-76ae135da058\"},{\"content\":{\"connectorIds\":[\"Out3\"],\"side\":\"TOP\"},\"type\":\"ConnectorPlacement.EquallySpacedRectSide\",\"uuid\":\"02c95e6b-ea4d-4952-978a-25b4914c2c12\"}]},\"type\":\"ConnectorPlacement.EquallySpacedConnector\",\"uuid\":\"3ff29f82-1f4c-432e-8c89-df3d4bc3a019\"}],\"packageUris\":[\"http://schema.mathworks.com/mf0/Connector/R2020b\"],\"version\":\"1.0\"}"
  Visualise F_spring : Subsystem  Commented=on
  Visualise Normal_Force : Subsystem  Commented=on
  Visualise sus disp : Subsystem  Commented=on
  Fz : Outport
  F_aero_down : Outport  Port=2
  Zs_static : Outport  Port=3
  Zs : Outport  Port=4
  wires:
  theta/1 -> Memory1/1
  phi/1 -> Memory2/1
  ARB/1(F_arb) -> MATLAB Function/1(F_arb)
  MATLAB Function/1(Fz) -> Visualise Normal_Force/1(F_z), Fz/1
  vel/1 -> MATLAB Function1/1(v)
  MATLAB Function1/1(F_aero_down) -> F_aero_down/1, Spring_forces/3(F_aero)
  Spring_forces/2(F_spring) -> MATLAB Function/2(F_spring), Visualise F_spring/1(F_spring)
  Spring_forces/1(Zs) -> Visualise sus disp/1(Zs), ARB/1(Zs), Zs/1
  Spring_forces/3(Zs1) -> Zs_static/1
  Memory1/1 -> Spring_forces/1(theta)
  Memory2/1 -> Spring_forces/2(phi)

== system vehicle_model_999/Rolling and Drag forces ==
  Fz : Inport
  Steer_FL : Inport  Port=2
  Steer_FR : Inport  Port=3
  vx : Inport  Port=4
  vy : Inport  Port=5
  Aero Drag : MATLAB Function  TreatAsAtomicUnit=on
  Bus Creator : BusCreator  Inputs=3
  MATLAB Function : MATLAB Function  TreatAsAtomicUnit=on
  Rolling Forces : MATLAB Function  TreatAsAtomicUnit=on
  Terminator : Terminator
  To Workspace : ToWorkspace  Commented=on  VariableName=Dragforce  SaveFormat=Timeseries  SampleTime=-1
  Roll_and_aero : Outport
  wires:
  Steer_FL/1 -> Rolling Forces/2(Steer_FL)
  vx/1 -> Aero Drag/1(vx)
  Fz/1 -> Rolling Forces/1(Fz)
  Aero Drag/1(B_F_aero) -> MATLAB Function/1(u), Bus Creator/3  "B_F_aero"
  Rolling Forces/1(Fx_rr_b) -> Bus Creator/1  "B_Fx_Roll"
  Steer_FR/1 -> Rolling Forces/3(Steer_FR)
  vy/1 -> Aero Drag/2(vy)
  Rolling Forces/2(Fy_rr_b) -> Bus Creator/2  "B_Fy_roll"
  Bus Creator/1 -> Roll_and_aero/1
  MATLAB Function/1(y) -> To Workspace/1, Terminator/1  "Drag_force"

== system vehicle_model_999/Steering Kinematics ==
  Steer_Input : Inport
  Ackermann_Pct : Inport  Port=2
  Bus Creator1 : BusCreator  Inputs=2
  Steering Kinematics : MATLAB Function  TreatAsAtomicUnit=on
  To Workspace : ToWorkspace  VariableName=steer_L  SaveFormat=Timeseries  SampleTime=-1
  To Workspace1 : ToWorkspace  VariableName=steer_R  SaveFormat=Timeseries  SampleTime=-1
  Steering Angles : Outport
  wires:
  Steering Kinematics/1(Steer_FL) -> To Workspace/1, Bus Creator1/1  "Steer_FL"
  Steer_Input/1 -> Steering Kinematics/1(Steer_Input)
  Steering Kinematics/2(Steer_FR) -> To Workspace1/1, Bus Creator1/2  "Steer_FR"
  Ackermann_Pct/1 -> Steering Kinematics/2(Ackermann_Pct)
  Bus Creator1/1 -> Steering Angles/1

== system vehicle_model_999/Subsystem ==
  toe : Inport
  slip_angles : Inport  Port=2
  Subtract : Sum  Inputs=+-
  Out1 : Outport
  wires:
  slip_angles/1 -> Subtract/1
  toe/1 -> Subtract/2
  Subtract/1 -> Out1/1

== system vehicle_model_999/Subsystem1 ==
  Vx : Inport
  Fx_ss : Inport  Port=2
  Integrator : Integrator
  MATLAB Function : MATLAB Function  TreatAsAtomicUnit=on
  Fx_w : Outport
  wires:
  Fx_ss/1 -> MATLAB Function/1(Fx_ss)
  MATLAB Function/1(Fx_dot) -> Integrator/1
  Integrator/1 -> Fx_w/1, MATLAB Function/2(Fx_act)
  Vx/1 -> MATLAB Function/3(Vx)

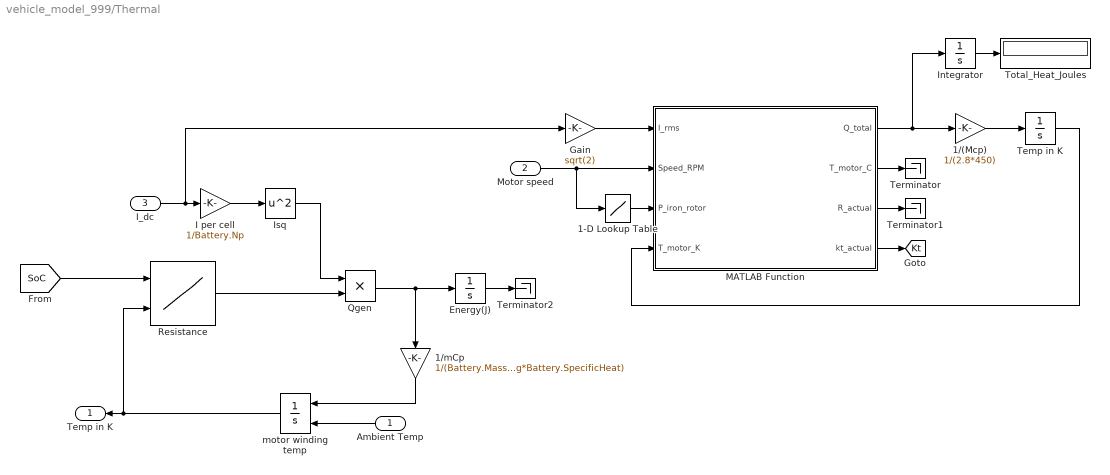
== system vehicle_model_999/Thermal ==
  Ambient Temp : Inport
  Motor speed : Inport  Port=2
  I_dc : Inport  Port=3
  1-D Lookup Table : Lookup_n-D  NumberOfTableDimensions=1  BreakpointsForDimension1=[0 5000 10000 12500 15000 20000]  Table=[0 105 230 300 310 315]  InternalRulePriority=Speed  RndMeth=Simplest
  1/(Mcp) : Gain  Gain=1/(2.8*450)
  1/mCp : Gain  Gain=1/(Battery.Mass_kg*Battery.SpecificHeat)
  Energy(J) : Integrator
  Gain : Gain  Gain=sqrt(2)
  I per cell : Gain  Gain=1/Battery.Np
  Integrator : Integrator
  Isq : Math  Operator=square
  MATLAB Function : MATLAB Function  TreatAsAtomicUnit=on
  Qgen : Product
  Resistance : Lookup_n-D  BreakpointsForDimension1=Battery.SoC_vec  BreakpointsForDimension2=Battery.T_vec  Table=Battery.R0_map+Battery.R1_map  InternalRulePriority=Speed  RndMeth=Simplest
      settings: InputPortMap=u0,u1
  "Temp in K " : Integrator  InitialCondition=293.15  LimitOutput=on  UpperSaturationLimit=423.15  LowerSaturationLimit=293.15
  Terminator : Terminator
  Terminator1 : Terminator
  Terminator2 : Terminator
  Total_Heat_Joules : Display
  motor winding temp : Integrator  InitialConditionSource=external  InitialCondition=298.15
  Temp in K : Outport
  tag scope: Kt=global
  wires:
  I_dc/1 -> Gain/1, I per cell/1
  MATLAB Function/2(T_motor_C) -> Terminator/1
  MATLAB Function/1(Q_total) -> Integrator/1, 1/(Mcp)/1
  1-D Lookup Table/1 -> MATLAB Function/3(P_iron_rotor)
  I per cell/1 -> Isq/1
  Energy(J)/1 -> Terminator2/1
  "Temp in K "/1 -> MATLAB Function/4(T_motor_K)
  Isq/1 -> Qgen/1
  MATLAB Function/3(R_actual) -> Terminator1/1
  [SoC] -> Resistance/1
  Motor speed/1 -> MATLAB Function/2(Speed_RPM), 1-D Lookup Table/1
  Gain/1 -> MATLAB Function/1(I_rms)
  Resistance/1 -> Qgen/2
  Integrator/1 -> Total_Heat_Joules/1
  1/(Mcp)/1 -> "Temp in K "/1
  Ambient Temp/1 -> motor winding temp/2
  Qgen/1 -> Energy(J)/1, 1/mCp/1
  motor winding temp/1 -> Temp in K/1, Resistance/2
  1/mCp/1 -> motor winding temp/1
  MATLAB Function/4(kt_actual) -> [Kt]

== system vehicle_model_999/Toe_including_compliances1 ==
  Fy : Inport
  Fx : Inport  Port=2
  Mz : Inport  Port=3
  Mux1 : Mux
  toe_fl1 : MATLAB Function  TreatAsAtomicUnit=on
  Out2 : Outport
  wires:
  Mux1/1 -> Out2/1
  Mz/1 -> toe_fl1/3(Mz)
  Fx/1 -> toe_fl1/2(Fx_tire)
  Fy/1 -> toe_fl1/1(Fy_tire)
  toe_fl1/1(Toe_fl) -> Mux1/1
  toe_fl1/2(Toe_fr) -> Mux1/2
  toe_fl1/3(Toe_rl) -> Mux1/3
  toe_fl1/4(Toe_rr) -> Mux1/4

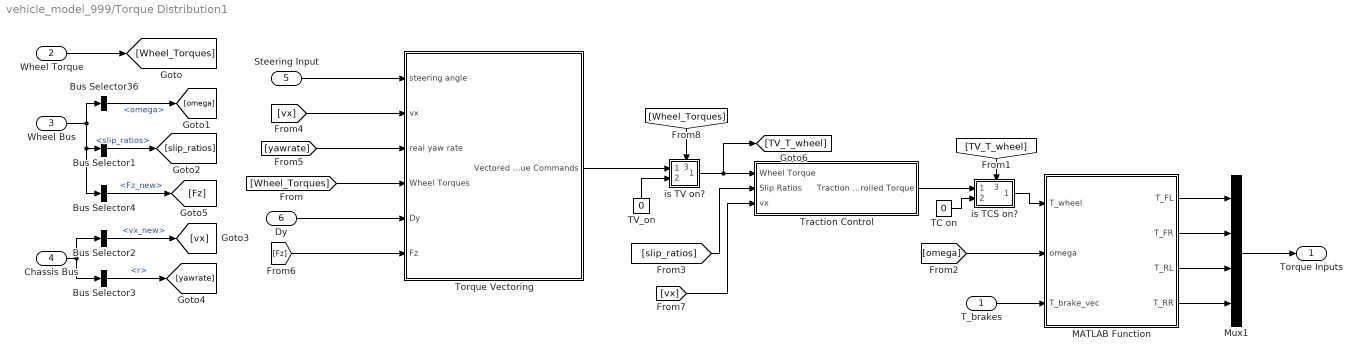
== system vehicle_model_999/Torque Distribution1 ==
  T_brakes : Inport
  Wheel Torque : Inport  Port=2
  Wheel Bus : Inport  Port=3
  Chassis Bus : Inport  Port=4
  Steering Input : Inport  Port=5
  Dy : Inport  Port=6
  Bus Selector1 : BusSelector  OutputSignals=slip_ratios
  Bus Selector2 : BusSelector  OutputSignals=vx_new
  Bus Selector3 : BusSelector  OutputSignals=r
  Bus Selector36 : BusSelector  OutputSignals=omega
  Bus Selector4 : BusSelector  OutputSignals=Fz_new
  MATLAB Function : MATLAB Function  TreatAsAtomicUnit=on
  Mux1 : Mux
  TC on : Constant  Value=0
  TV_on : Constant  Value=0
  Torque Vectoring : Subsystem
  Traction Control : Subsystem
  is TCS on? : Subsystem
      settings: PortSchema="{\"entries\":[{\"content\":{\"sides\":[{\"content\":{\"connectorIds\":[\"In1\",\"In2\"]},\"type\":\"ConnectorPlacement.EquallySpacedRectSide\",\"uuid\":\"dc8df3c8-a53f-4de0-9df1-c7ce6985ad6f\"},{\"content\":{\"connectorIds\":[\"Out1\"],\"side\":\"RIGHT\"},\"type\":\"ConnectorPlacement.EquallySpacedRectSide\",\"uuid\":\"042501be-c855-4a6a-885a-a96d559db999\"},{\"content\":{\"connectorIds\":[\"In3\"],\"side\":\"TOP\"},\"type\":\"ConnectorPlacement.EquallySpacedRectSide\",\"uuid\":\"e6b24d4f-1e31-4513-950e-4f31e3010837\"}]},\"type\":\"ConnectorPlacement.EquallySpacedConnector\",\"uuid\":\"efc7ad52-73a3-41d4-9bb0-a43132bb4628\"}],\"packageUris\":[\"http://schema.mathworks.com/mf0/Connector/R2020b\"],\"version\":\"1.0\"}"
  is TV on? : Subsystem
      settings: PortSchema="{\"entries\":[{\"content\":{\"sides\":[{\"content\":{\"connectorIds\":[\"In1\",\"In2\"]},\"type\":\"ConnectorPlacement.EquallySpacedRectSide\",\"uuid\":\"dc8df3c8-a53f-4de0-9df1-c7ce6985ad6f\"},{\"content\":{\"connectorIds\":[\"Out1\"],\"side\":\"RIGHT\"},\"type\":\"ConnectorPlacement.EquallySpacedRectSide\",\"uuid\":\"042501be-c855-4a6a-885a-a96d559db999\"},{\"content\":{\"connectorIds\":[\"In3\"],\"side\":\"TOP\"},\"type\":\"ConnectorPlacement.EquallySpacedRectSide\",\"uuid\":\"e6b24d4f-1e31-4513-950e-4f31e3010837\"},{\"content\":{\"side\":\"BOTTOM\"},\"type\":\"ConnectorPlacement.EquallySpacedRectSide\",\"uuid\":\"10630930-7341-43aa-b9d4-dad8f31a30ac\"}]},\"type\":\"ConnectorPlacement.EquallySpacedConnector\",\"uuid\":\"efc7ad52-73a3-41d4-9bb0-a43132bb4628\"}],\"packageUris\":[\"http://schema.mathworks.com/mf0/Connector/R2020b\"],\"version\":\"1.0\"}"
  Torque Inputs : Outport
  wires:
  T_brakes/1 -> MATLAB Function/3(T_brake_vec)
  MATLAB Function/1(T_FL) -> Mux1/1
  MATLAB Function/2(T_FR) -> Mux1/2
  MATLAB Function/3(T_RL) -> Mux1/3
  MATLAB Function/4(T_RR) -> Mux1/4
  Mux1/1 -> Torque Inputs/1
  Wheel Bus/1 -> Bus Selector36/1, Bus Selector4/1, Bus Selector1/1
  Chassis Bus/1 -> Bus Selector3/1, Bus Selector2/1
  Wheel Torque/1 -> [Wheel_Torques]
  [Wheel_Torques] -> Torque Vectoring/4(Wheel Torques)
  Bus Selector36/1 -> [omega]  "<omega>"
  [omega] -> MATLAB Function/2(omega)
  Bus Selector1/1 -> [slip_ratios]  "<slip_ratios>"
  [slip_ratios] -> Traction Control/2(Slip Ratios)
  [vx] -> Torque Vectoring/2(vx)
  Bus Selector2/1 -> [vx]  "<vx_new>"
  Bus Selector3/1 -> [yawrate]  "<r>"
  [yawrate] -> Torque Vectoring/3(real yaw rate)
  Steering Input/1 -> Torque Vectoring/1(steering angle)
  is TCS on?/1(torque_output) -> MATLAB Function/1(T_wheel)
  Bus Selector4/1 -> [Fz]  "<Fz_new>"
  Dy/1 -> Torque Vectoring/5(Dy)
  [Fz] -> Torque Vectoring/6(Fz)
  [vx] -> Traction Control/3(vx)
  Torque Vectoring/1(Vectored Torque Commands) -> is TV on?/1(vectored_torque)
  is TV on?/1(torque_output) -> Traction Control/1(Wheel Torque), [TV_T_wheel]
  [Wheel_Torques] -> is TV on?/3(wheel_torque)
  Traction Control/1(Traction Controlled Torque) -> is TCS on?/1(traction_controlled_torque)
  [TV_T_wheel] -> is TCS on?/3(TV_T_wheel)
  TC on/1 -> is TCS on?/2(In1)
  TV_on/1 -> is TV on?/2(In1)

== system vehicle_model_999/Visualise slip_angles ==
  slip_angles : Inport
  MATLAB Function : MATLAB Function  TreatAsAtomicUnit=on
  To Workspace : ToWorkspace  VariableName=slip_angle_fl  SaveFormat=Timeseries  SampleTime=-1
  To Workspace1 : ToWorkspace  VariableName=slip_angle_fr  SaveFormat=Timeseries  SampleTime=-1
  To Workspace2 : ToWorkspace  VariableName=slip_angle_rl  SaveFormat=Timeseries  SampleTime=-1
  To Workspace3 : ToWorkspace  VariableName=slip_angle_rr  SaveFormat=Timeseries  SampleTime=-1
  Visualise slip_angle : Scope  NumInputPorts=4
      settings: ActiveDisplayYMinimum=-1  ActiveDisplayYMaximum=1  DataLoggingVariableName=ScopeData3
  wires:
  MATLAB Function/4(alpha_rr) -> To Workspace3/1, Visualise slip_angle/4  "alpha_rr"
  MATLAB Function/3(alpha_rl) -> To Workspace2/1, Visualise slip_angle/3  "alpha_rl"
  MATLAB Function/2(alpha_fr) -> To Workspace1/1, Visualise slip_angle/2  "alpha_fr"
  MATLAB Function/1(alpha_fl) -> To Workspace/1, Visualise slip_angle/1  "alpha_fl"
  slip_angles/1 -> MATLAB Function/1(slip_angles)

== system vehicle_model_999/Visualise slip_ratios ==
  slip_ratio : Inport
  MATLAB Function : MATLAB Function  TreatAsAtomicUnit=on
  To Workspace : ToWorkspace  VariableName=slip_ratio_fl  SaveFormat=Timeseries  SampleTime=-1
  To Workspace1 : ToWorkspace  VariableName=slip_ratio_fr  SaveFormat=Timeseries  SampleTime=-1
  To Workspace2 : ToWorkspace  VariableName=slip_ratio_rl  SaveFormat=Timeseries  SampleTime=-1
  To Workspace3 : ToWorkspace  VariableName=slip_ratio_rr  SaveFormat=Timeseries  SampleTime=-1
  Visualise slip_ratio : Scope  NumInputPorts=4
      settings: ActiveDisplayYMinimum=-0.0042686362260250313  ActiveDisplayYMaximum=-0.0025424073705559666  DataLoggingVariableName=ScopeData3
  wires:
  slip_ratio/1 -> MATLAB Function/1(slip_ratio)
  MATLAB Function/1(SR_fl) -> Visualise slip_ratio/1, To Workspace/1  "slip_ratio_fl"
  MATLAB Function/2(SR_fr) -> Visualise slip_ratio/2, To Workspace1/1  "slip_ratio_fr"
  MATLAB Function/3(SR_rl) -> Visualise slip_ratio/3, To Workspace2/1  "slip_ratio_rl"
  MATLAB Function/4(SR_rr) -> Visualise slip_ratio/4, To Workspace3/1  "slip_ratio_rr"

== system vehicle_model_999/Visualise_Fx_tire ==
  Fx_tire : Inport
  MATLAB Function : MATLAB Function  TreatAsAtomicUnit=on
  To Workspace : ToWorkspace  VariableName=Fx_fl  SaveFormat=Timeseries  SampleTime=-1
  To Workspace1 : ToWorkspace  VariableName=Fx_fr  SaveFormat=Timeseries  SampleTime=-1
  To Workspace2 : ToWorkspace  VariableName=Fx_rl  SaveFormat=Timeseries  SampleTime=-1
  To Workspace3 : ToWorkspace  VariableName=Fx_rr  SaveFormat=Timeseries  SampleTime=-1
  Visualise Fx tire : Scope  NumInputPorts=4
      settings: ActiveDisplayYMinimum=-157.0903  ActiveDisplayYMaximum=17.4645  DataLoggingVariableName=ScopeData4
  wires:
  Fx_tire/1 -> MATLAB Function/1(Fx_tire)
  MATLAB Function/1(Fx_fl) -> To Workspace/1, Visualise Fx tire/1  "Fx_fl"
  MATLAB Function/2(Fx_fr) -> Visualise Fx tire/2, To Workspace1/1  "Fx_fr"
  MATLAB Function/3(Fx_rl) -> Visualise Fx tire/3, To Workspace2/1  "Fx_rl"
  MATLAB Function/4(Fx_rr) -> Visualise Fx tire/4, To Workspace3/1  "Fx_rr"

== system vehicle_model_999/Visualise_Fx_tire1 ==
  Fz_tire : Inport
  MATLAB Function : MATLAB Function  TreatAsAtomicUnit=on
  To Workspace : ToWorkspace  VariableName=Fz_fl  SaveFormat=Timeseries  SampleTime=-1
  To Workspace1 : ToWorkspace  VariableName=Fz_fr  SaveFormat=Timeseries  SampleTime=-1
  To Workspace2 : ToWorkspace  VariableName=Fz_rl  SaveFormat=Timeseries  SampleTime=-1
  To Workspace3 : ToWorkspace  VariableName=Fz_rr  SaveFormat=Timeseries  SampleTime=-1
  Visualise Fz tire : Scope  Commented=on  NumInputPorts=4
  wires:
  MATLAB Function/4(Fz_rr) -> To Workspace3/1, Visualise Fz tire/4  "Fz_rr"
  MATLAB Function/3(Fz_rl) -> To Workspace2/1, Visualise Fz tire/3  "Fz_rl"
  MATLAB Function/2(Fz_fr) -> To Workspace1/1, Visualise Fz tire/2  "Fz_fr"
  MATLAB Function/1(Fz_fl) -> To Workspace/1, Visualise Fz tire/1  "Fz_fl"
  Fz_tire/1 -> MATLAB Function/1(Fz_tire)

== system vehicle_model_999/Visualise_Fy_B ==
  Fy_B : Inport
  MATLAB Function : MATLAB Function  TreatAsAtomicUnit=on
  Visualise Fy_B : Scope  Commented=on  NumInputPorts=4
  wires:
  Fy_B/1 -> MATLAB Function/1(Fy_tire)
  MATLAB Function/2(Fy_B_fr) -> Visualise Fy_B/2  "Fy_B_fr"
  MATLAB Function/4(Fy_B_rr) -> Visualise Fy_B/4  "Fy_B_rr"
  MATLAB Function/1(Fy_B_fl) -> Visualise Fy_B/1  "Fy_B_fl"
  MATLAB Function/3(Fy_B_rl) -> Visualise Fy_B/3  "Fy_B_rl"

== system vehicle_model_999/Visualise_Fy_tire ==
  Fy_tire : Inport
  MATLAB Function : MATLAB Function  TreatAsAtomicUnit=on
  To Workspace : ToWorkspace  VariableName=Fy_fl  SaveFormat=Timeseries  SampleTime=-1
  To Workspace1 : ToWorkspace  VariableName=Fy_fr  SaveFormat=Timeseries  SampleTime=-1
  To Workspace2 : ToWorkspace  VariableName=Fy_rl  SaveFormat=Timeseries  SampleTime=-1
  To Workspace3 : ToWorkspace  VariableName=Fy_rr  SaveFormat=Timeseries  SampleTime=-1
  Visualise Fy tire : Scope  NumInputPorts=4
      settings: ActiveDisplayYMinimum=-577.98244716833722  ActiveDisplayYMaximum=1065.6680014876922
  wires:
  Fy_tire/1 -> MATLAB Function/1(Fy_tire)
  MATLAB Function/2(Fy_fr) -> Visualise Fy tire/2, To Workspace1/1  "Fy_fr"
  MATLAB Function/4(Fy_rr) -> Visualise Fy tire/4, To Workspace3/1  "Fy_rr"
  MATLAB Function/1(Fy_fl) -> Visualise Fy tire/1, To Workspace/1  "Fy_fl"
  MATLAB Function/3(Fy_rl) -> Visualise Fy tire/3, To Workspace2/1  "Fy_rl"

== system vehicle_model_999/Visualiser ==
  mz : Inport
  mu_x : Inport  Port=2
  mu_y : Inport  Port=3
  Demux : Demux
  Demux1 : Demux
  Demux2 : Demux
  Scope : Scope  NumInputPorts=4
  Scope1 : Scope  NumInputPorts=4
  Scope2 : Scope  NumInputPorts=4
  wires:
  mz/1 -> Demux/1
  Demux/1 -> Scope/1
  Demux/2 -> Scope/2
  Demux/3 -> Scope/3
  Demux/4 -> Scope/4
  Demux1/3 -> Scope1/3
  Demux1/2 -> Scope1/2
  mu_x/1 -> Demux1/1
  Demux1/1 -> Scope1/1
  Demux1/4 -> Scope1/4
  Demux2/3 -> Scope2/3
  Demux2/2 -> Scope2/2
  mu_y/1 -> Demux2/1
  Demux2/1 -> Scope2/1
  Demux2/4 -> Scope2/4

== system vehicle_model_999/Wheel Dynamics ==
  T_in : Inport
  Fx : Inport  Port=2
  Omega : Inport  Port=3
  Fx_tire : Inport  Port=4
  Integrator : Integrator  InitialCondition=init_vx/Par.R0  LimitOutput=on  UpperSaturationLimit=1e6
  MATLAB Function : MATLAB Function  TreatAsAtomicUnit=on
  omega : Outport
  wires:
  Integrator/1 -> omega/1
  T_in/1 -> MATLAB Function/1(T_in)
  Fx/1 -> MATLAB Function/2(Fx_rr)
  Omega/1 -> MATLAB Function/4(Omega)
  MATLAB Function/1(Omega_dot) -> Integrator/1
  Fx_tire/1 -> MATLAB Function/3(Fx_tire)

== system vehicle_model_999/brake_input_simulink ==
  Clock : Clock
  Constant : Constant
  Constant1 : Constant  Value=0
  Switch : Switch  Criteria=u2 > Threshold  Threshold=2  SaturateOnIntegerOverflow=off  InputSameDT=off
  brake_sim : Outport
  wires:
  Clock/1 -> Switch/2
  Constant/1 -> Switch/1
  Constant1/1 -> Switch/3
  Switch/1 -> brake_sim/1

== system vehicle_model_999/input_select ==
  brake_sim : Inport
  vel : Inport  Port=2
  Brake Variant Subsystem : Subsystem  Variant=on
  Brake pedal : Outport
  accln_for_map1 : Outport  Port=2
  wires:
  Brake Variant Subsystem/1(brake_input) -> Brake pedal/1
  brake_sim/1 -> Brake Variant Subsystem/1(brake_sim)
  vel/1 -> Brake Variant Subsystem/2(vel)
  Brake Variant Subsystem/2(accln) -> accln_for_map1/1

== system vehicle_model_999/input_selection ==
  In1 : Inport
  Steering Variant Subsystem : Subsystem  Variant=on
  Steer Input : Outport
  wires:
  Steering Variant Subsystem/1(Steer Input) -> Steer Input/1
  In1/1 -> Steering Variant Subsystem/1(In1)
